simulink model "firefighting_drone_2"  (R2022b)
settings: Solver=FixedStepAuto  StartTime=0.0  StopTime=80  FixedStep=0.1  RelTol=1e-3
(part 1 of 4)
settings Model: Creator=User  LastModifiedBy=hugoaraujo
settings SolverCC: AlgebraicLoopSolver=TrustRegion
settings DataIOCC: ReturnWorkspaceOutputs=off
settings DebuggingCC: UnconnectedInputMsg=warning  UnconnectedOutputMsg=warning  UnconnectedLineMsg=warning  SFMachineParentedDataDiag=warning  ArithmeticOperatorsInVariantConditions=warning
settings ModelReferenceCC: EnableRefExpFcnMdlSchedulingChecks=on
settings SFSimCC: SimUseLocalCustomCode=off  CustomCodeUndefinedFunction=UseInterfaceOnly
settings RTWCC: RTWUseLocalCustomCode=off  DLArmComputeVersion=19.05
settings CodeAppCC: StateflowObjectComments=on

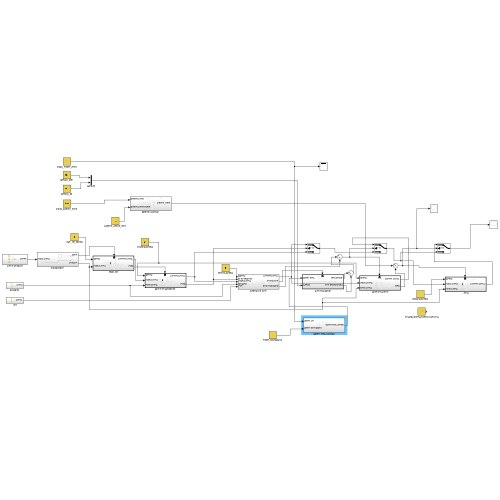
[thumbnail: Simulink's stored preview of the top-level diagram]
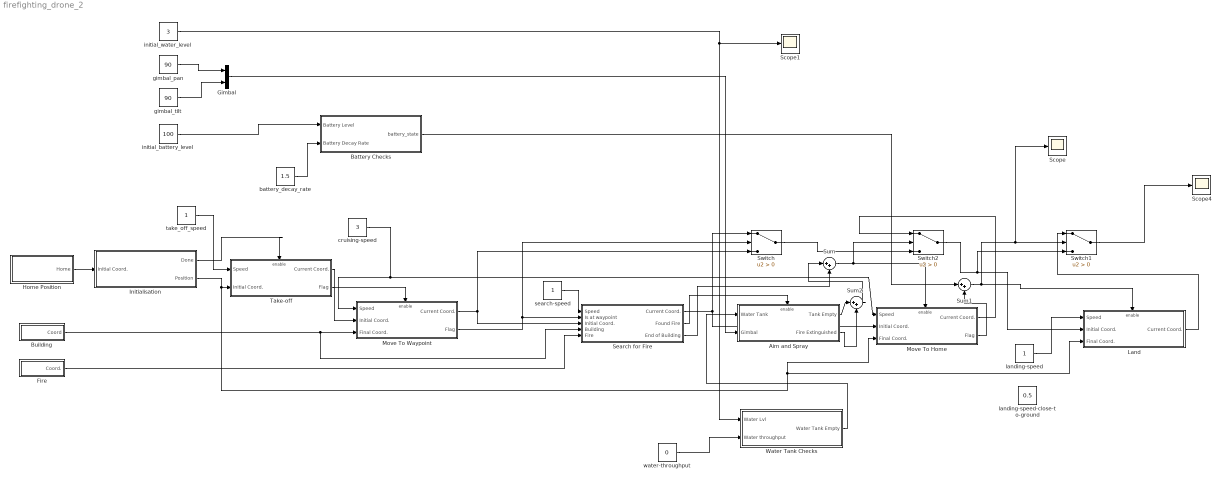
== system firefighting_drone_2 ==
  Aim and Spray : Subsystem
  Battery Checks : Subsystem
  Building : Subsystem
  Fire : Subsystem
  Gimbal : Mux  Inputs=2
  Home Position : Subsystem
  Initialisation : Subsystem
  Land : Subsystem
  Move To Home : Subsystem
  Move To Waypoint : Subsystem
  Scope : Scope
  Scope1 : Scope
  Scope4 : Scope
  Search for Fire : Subsystem
  Sum : Sum  Inputs=|++
  Sum1 : Sum  Inputs=|++
  Sum2 : Sum  Inputs=|++
  Switch : Switch  Criteria=u2 > Threshold  SaturateOnIntegerOverflow=off  InputSameDT=off
  Switch1 : Switch  Criteria=u2 > Threshold  SaturateOnIntegerOverflow=off  InputSameDT=off
  Switch2 : Switch  Criteria=u2 > Threshold  SaturateOnIntegerOverflow=off  InputSameDT=off
  Take-off : Subsystem
  Water Tank Checks : Subsystem
  battery_decay_rate : Constant  Value=1.5
  cruising-speed : Constant  Value=3
  gimbal_pan : Constant  Value=90
  gimbal_tilt : Constant  Value=90
  initial_battery_level : Constant  Value=100
  initial_water_level : Constant  Value=3
  landing-speed : Constant
  landing-speed-close-to-ground : Constant  Value=0.5
  search-speed : Constant
  take_off_speed : Constant
  water-throughput : Constant  Value=0
  wires:
  Building/1(Coord) -> Search for Fire/4(Building), Move To Waypoint/3(Final Coord.)
  cruising-speed/1 -> Move To Waypoint/1(Speed), Move To Home/1(Speed)
  Move To Waypoint/2(Flag) -> Switch/2, Search for Fire/2(Is at waypoint)
  Move To Waypoint/1(Current Coord.) -> Search for Fire/3(Initial Coord.), Switch/3
  Sum/1 -> Move To Home/Enable, Switch2/2
  Switch/1 -> Switch2/3
  Move To Home/1(Current Coord.) -> Switch2/1
  Take-off/2(Flag) -> Move To Waypoint/Enable
  Take-off/1(Current Coord.) -> Move To Waypoint/2(Initial Coord.)
  battery_decay_rate/1 -> Battery Checks/2(Battery Decay Rate)
  initial_battery_level/1 -> Battery Checks/1(Battery Level)
  gimbal_pan/1 -> Gimbal/1
  gimbal_tilt/1 -> Gimbal/2
  Battery Checks/1(battery_state) -> Sum1/1
  Move To Home/2(Flag) -> Sum1/2
  Sum1/1 -> Land/Enable, Scope/1, Switch1/2
  Initialisation/2(Position) -> Move To Home/3(Final Coord.), Land/3(Final Coord.), Take-off/2(Initial Coord.)
  Search for Fire/1(Current Coord.) -> Move To Home/2(Initial Coord.), Switch/1
  Fire/1(Coord.) -> Search for Fire/5(Fire)
  Search for Fire/2(Found Fire) -> Aim and Spray/Enable
  Search for Fire/3(End of Building) -> Sum/2
  Initialisation/1(Done) -> Take-off/Enable
  Home Position/1(Home) -> Initialisation/1(Initial Coord.)
  search-speed/1 -> Search for Fire/1(Speed)
  Switch2/1 -> Land/2(Initial Coord.), Switch1/3
  landing-speed/1 -> Land/1(Speed)
  Water Tank Checks/1(Water Tank Empty) -> Aim and Spray/1(Water Tank)
  Gimbal/1 -> Aim and Spray/2(Gimbal)
  initial_water_level/1 -> Scope1/1, Water Tank Checks/1(Water Lvl)
  Land/1(Current Coord.) -> Switch1/1
  Switch1/1 -> Scope4/1
  take_off_speed/1 -> Take-off/1(Speed)
  water-throughput/1 -> Water Tank Checks/2(Water throughput)
  Aim and Spray/2(Fire Extinguished) -> Sum2/2
  Aim and Spray/1(Tank Empty) -> Sum2/1
  Sum2/1 -> Sum/1

== system firefighting_drone_2/Aim and Spray ==
  Water Tank : Inport
  Gimbal : Inport  Port=2
  Enable : EnablePort
  Tank Empty : Outport
  Fire Extinguished : Outport  Port=2
  wires:
  Water Tank/1 -> Fire Extinguished/1, Tank Empty/1

== system firefighting_drone_2/Battery Checks ==
  Battery Level : Inport
  Battery Decay Rate : Inport  Port=2
  Constant : Constant  Value=0
  Constant1 : Constant  Value=2
  Constant2 : Constant
  If : If  IfExpression=u1 > 30  ElseIfExpressions=u1 > 15
  If Action Subsystem : Subsystem  TreatAsAtomicUnit=on
  If Action Subsystem1 : Subsystem  TreatAsAtomicUnit=on
  If Action Subsystem2 : Subsystem  TreatAsAtomicUnit=on
  Integrator : Integrator
  Merge : Merge  Inputs=3
  Scope : Scope
  Scope1 : Scope
  Sum2 : Sum  Inputs=|+-
  battery_state : Outport
  wires:
  Battery Decay Rate/1 -> Integrator/1
  Integrator/1 -> Sum2/2
  Battery Level/1 -> Sum2/1
  Sum2/1 -> Scope1/1, If/1
  Constant1/1 -> If Action Subsystem1/1(In1)
  If/1 -> If Action Subsystem/Action
  Constant/1 -> If Action Subsystem/1(In1)
  If Action Subsystem/1(Out1) -> Merge/1
  If Action Subsystem1/1(Out1) -> Merge/3
  Merge/1 -> Scope/1, battery_state/1
  If/3 -> If Action Subsystem1/Action
  Constant2/1 -> If Action Subsystem2/1(In1)
  If/2 -> If Action Subsystem2/Action
  If Action Subsystem2/1(Out1) -> Merge/2

== system firefighting_drone_2/Building ==
  Building.x : Constant  Value=25
  Building.y : Constant  Value=15
  Building.z : Constant  Value=2
  Mux : Mux  Inputs=3
  Coord : Outport  VectorParamsAs1DForOutWhenUnconnected=off
  wires:
  Building.y/1 -> Mux/2
  Building.z/1 -> Mux/3
  Building.x/1 -> Mux/1
  Mux/1 -> Coord/1

== system firefighting_drone_2/Fire ==
  Fire.x : Constant  Value=25
  Fire.y : Constant  Value=20
  Fire.z : Constant  Value=12
  Mux : Mux  Inputs=3
  Coord. : Outport  VectorParamsAs1DForOutWhenUnconnected=off
  wires:
  Fire.y/1 -> Mux/2
  Fire.z/1 -> Mux/3
  Fire.x/1 -> Mux/1
  Mux/1 -> Coord./1

== system firefighting_drone_2/Home Position ==
  Home.x : Constant  Value=0
  Home.y : Constant  Value=0
  Home.z : Constant  Value=0
  Mux : Mux  Inputs=3
  Home : Outport  VectorParamsAs1DForOutWhenUnconnected=off
  wires:
  Home.x/1 -> Mux/1
  Home.y/1 -> Mux/2
  Home.z/1 -> Mux/3
  Mux/1 -> Home/1

== system firefighting_drone_2/Initialisation ==
  Initial Coord. : Inport
  Constant : Constant
  Done : Outport  VectorParamsAs1DForOutWhenUnconnected=off
  Position : Outport  Port=2  VectorParamsAs1DForOutWhenUnconnected=off
  wires:
  Initial Coord./1 -> Position/1
  Constant/1 -> Done/1

== system firefighting_drone_2/Land ==
  Speed : Inport
  Initial Coord. : Inport  Port=2
  Final Coord. : Inport  Port=3
  Enable : EnablePort
  Constant : Constant
  Constant1 : Constant  Value=0
  Demux : Demux  Outputs=3
  Demux1 : Demux  Outputs=3
  Display : Display
  Display2 : Display
  Move Arm1 : Subsystem
  Move Arm2 : Subsystem
  Move Arm3 : Subsystem
  Mux : Mux  Inputs=3
  Mux1 : Mux  Inputs=3
  Scope : Scope
  Scope1 : Scope  NumInputPorts=3
  Scope2 : Scope
  Scope3 : Scope
  Sum : Sum  Inputs=3
  Switch : Switch  Threshold=3  SaturateOnIntegerOverflow=off  InputSameDT=off
  Current Coord. : Outport  VectorParamsAs1DForOutWhenUnconnected=off
  wires:
  Demux1/1 -> Mux1/1, Scope3/1, Move Arm1/3(Desired Angle)
  Demux/1 -> Scope2/1, Move Arm1/2(Starting Angle)
  Move Arm3/1(Out1) -> Scope1/3, Mux/3  "Z"
  Demux/2 -> Move Arm2/2(Starting Angle)
  Speed/1 -> Move Arm2/1(Angular Accel), Move Arm3/1(Angular Accel), Move Arm1/1(Angular Accel)
  Move Arm2/1(Out1) -> Mux/2, Scope1/2  "Y"
  Move Arm1/1(Out1) -> Mux/1, Scope1/1  "X"
  Demux/3 -> Move Arm3/2(Starting Angle)
  Demux1/2 -> Move Arm2/3(Desired Angle), Mux1/2
  Demux1/3 -> Move Arm3/3(Desired Angle), Mux1/3
  Mux/1 -> Display2/1, Current Coord./1, Scope/1
  Mux1/1 -> Display/1
  Initial Coord./1 -> Demux/1
  Final Coord./1 -> Demux1/1
  Move Arm3/2(Done) -> Sum/3
  Move Arm1/2(Done) -> Sum/1
  Move Arm2/2(Done) -> Sum/2
  Constant1/1 -> Switch/3
  Constant/1 -> Switch/1
  Sum/1 -> Switch/2
  Switch/1 -> ?

== system firefighting_drone_2/Move To Home ==
  Speed : Inport
  Initial Coord. : Inport  Port=2
  Final Coord. : Inport  Port=3
  Enable : EnablePort
  Constant : Constant
  Constant1 : Constant  Value=0
  Demux : Demux  Outputs=3
  Demux1 : Demux  Outputs=3
  Display : Display
  Display2 : Display
  Move Arm1 : Subsystem
  Move Arm2 : Subsystem
  Move Arm3 : Subsystem
  Mux : Mux  Inputs=3
  Mux1 : Mux  Inputs=3
  Scope : Scope
  Scope1 : Scope  NumInputPorts=3
  Scope2 : Scope
  Scope3 : Scope
  Sum : Sum  Inputs=3
  Switch : Switch  Threshold=3  SaturateOnIntegerOverflow=off  InputSameDT=off
  Current Coord. : Outport  VectorParamsAs1DForOutWhenUnconnected=off
  Flag : Outport  Port=2  VectorParamsAs1DForOutWhenUnconnected=off
  wires:
  Demux1/1 -> Mux1/1, Scope3/1, Move Arm1/3(Desired Angle)
  Demux/1 -> Scope2/1, Move Arm1/2(Starting Angle)
  Move Arm3/1(Out1) -> Scope1/3, Mux/3  "Z"
  Demux/2 -> Move Arm2/2(Starting Angle)
  Speed/1 -> Move Arm2/1(Angular Accel), Move Arm3/1(Angular Accel), Move Arm1/1(Angular Accel)
  Move Arm2/1(Out1) -> Mux/2, Scope1/2  "Y"
  Move Arm1/1(Out1) -> Mux/1, Scope1/1  "X"
  Demux/3 -> Move Arm3/2(Starting Angle)
  Demux1/2 -> Move Arm2/3(Desired Angle), Mux1/2
  Demux1/3 -> Move Arm3/3(Desired Angle), Mux1/3
  Mux/1 -> Display2/1, Current Coord./1, Scope/1
  Mux1/1 -> Display/1
  Initial Coord./1 -> Demux/1
  Final Coord./1 -> Demux1/1
  Move Arm3/2(Done) -> Sum/3
  Move Arm1/2(Done) -> Sum/1
  Move Arm2/2(Done) -> Sum/2
  Constant1/1 -> Switch/3
  Constant/1 -> Switch/1
  Sum/1 -> Switch/2
  Switch/1 -> Flag/1

== system firefighting_drone_2/Move To Waypoint ==
  Speed : Inport
  Initial Coord. : Inport  Port=2
  Final Coord. : Inport  Port=3
  Enable : EnablePort
  Constant : Constant
  Constant1 : Constant  Value=0
  Demux : Demux  Outputs=3
  Demux1 : Demux  Outputs=3
  Display : Display
  Display2 : Display
  Move X : Subsystem
  Move Y : Subsystem
  Move Z : Subsystem
  Mux : Mux  Inputs=3
  Mux1 : Mux  Inputs=3
  Scope : Scope
  Scope1 : Scope  NumInputPorts=3
  Scope2 : Scope
  Scope3 : Scope
  Sum : Sum  Inputs=3
  Switch : Switch  Threshold=3  SaturateOnIntegerOverflow=off  InputSameDT=off
  Current Coord. : Outport  VectorParamsAs1DForOutWhenUnconnected=off
  Flag : Outport  Port=2  VectorParamsAs1DForOutWhenUnconnected=off
  wires:
  Demux1/1 -> Mux1/1, Scope3/1, Move X/3(Desired Angle)
  Demux/1 -> Scope2/1, Move X/2(Starting Angle)
  Move Z/1(Out1) -> Scope1/3, Mux/3
  Demux/2 -> Move Y/2(Starting Angle)
  Speed/1 -> Move Y/1(Angular Accel), Move Z/1(Angular Accel), Move X/1(Angular Accel)
  Move Y/1(Out1) -> Mux/2, Scope1/2
  Move X/1(Out1) -> Mux/1, Scope1/1
  Demux/3 -> Move Z/2(Starting Angle)
  Demux1/2 -> Move Y/3(Desired Angle), Mux1/2
  Demux1/3 -> Move Z/3(Desired Angle), Mux1/3
  Mux/1 -> Display2/1, Current Coord./1, Scope/1
  Mux1/1 -> Display/1
  Initial Coord./1 -> Demux/1
  Final Coord./1 -> Demux1/1
  Move Z/2(Done) -> Sum/3
  Move X/2(Done) -> Sum/1
  Move Y/2(Done) -> Sum/2
  Constant1/1 -> Switch/3
  Constant/1 -> Switch/1
  Sum/1 -> Switch/2
  Switch/1 -> Flag/1

== system firefighting_drone_2/Search for Fire ==
  Speed : Inport
  Is at waypoint : Inport  Port=2
  Initial Coord. : Inport  Port=3
  Building : Inport  Port=4
  Fire : Inport  Port=5
  Scope : Scope
  Seaerch-fire : Subsystem
  Current Coord. : Outport
  Found Fire : Outport  Port=2
  End of Building : Outport  Port=3
  wires:
  Seaerch-fire/3(Flag1) -> End of Building/1
  Seaerch-fire/2(Flag) -> Scope/1, Found Fire/1
  Seaerch-fire/1(Current Coord.) -> Current Coord./1
  Building/1 -> Seaerch-fire/4(Building)
  Is at waypoint/1 -> Seaerch-fire/Enable
  Fire/1 -> Seaerch-fire/3(Fire)
  Speed/1 -> Seaerch-fire/1(Speed)
  Initial Coord./1 -> Seaerch-fire/2(Initial Coord.)

== system firefighting_drone_2/Take-off ==
  Speed : Inport
  Initial Coord. : Inport  Port=2
  Enable : EnablePort
  Constant : Constant
  Constant1 : Constant  Value=0
  CoordX : Subsystem
  CoordY : Subsystem
  CoordZ : Subsystem
  Demux : Demux  Outputs=3
  Demux1 : Demux  Outputs=3
  Display : Display
  Display2 : Display
  Mux : Mux  Inputs=3
  Mux1 : Mux  Inputs=3
  Scope : Scope
  Scope1 : Scope  NumInputPorts=3
  Scope2 : Scope
  Scope3 : Scope
  Sum : Sum  Inputs=3
  Switch : Switch  Threshold=3  SaturateOnIntegerOverflow=off  InputSameDT=off
  Take-off Height : Subsystem
  Current Coord. : Outport  VectorParamsAs1DForOutWhenUnconnected=off
  Flag : Outport  Port=2  VectorParamsAs1DForOutWhenUnconnected=off
  wires:
  Demux1/1 -> Mux1/1, Scope3/1, CoordX/3(Desired Angle)
  Demux/1 -> Scope2/1, CoordX/2(Starting Angle)
  CoordZ/1(Out1) -> Scope1/3, Mux/3
  Demux/2 -> CoordY/2(Starting Angle)
  Speed/1 -> CoordY/1(Angular Accel), CoordZ/1(Angular Accel), CoordX/1(Angular Accel)
  CoordY/1(Out1) -> Mux/2, Scope1/2
  CoordX/1(Out1) -> Mux/1, Scope1/1
  Demux/3 -> CoordZ/2(Starting Angle)
  Demux1/2 -> CoordY/3(Desired Angle), Mux1/2
  Demux1/3 -> CoordZ/3(Desired Angle), Mux1/3
  Mux/1 -> Display2/1, Current Coord./1, Scope/1
  Mux1/1 -> Display/1
  Initial Coord./1 -> Demux/1
  Take-off Height/1(Coord) -> Demux1/1
  CoordZ/2(Done) -> Sum/3
  CoordX/2(Done) -> Sum/1
  CoordY/2(Done) -> Sum/2
  Constant1/1 -> Switch/3
  Constant/1 -> Switch/1
  Sum/1 -> Switch/2
  Switch/1 -> Flag/1

== system firefighting_drone_2/Water Tank Checks ==
  Water Lvl : Inport
  Water throughput : Inport  Port=2
  Constant2 : Constant  Value=0
  Constant3 : Constant
  If Action Subsystem : Subsystem  TreatAsAtomicUnit=on
  If Action Subsystem1 : Subsystem  TreatAsAtomicUnit=on
  If1 : If  IfExpression=u1 > 15
  Integrator : Integrator
  Merge : Merge
  Scope : Scope
  Sum2 : Sum  Inputs=|+-
  Water Tank Empty : Outport
  wires:
  Water throughput/1 -> Integrator/1
  Integrator/1 -> Sum2/2
  Water Lvl/1 -> Sum2/1
  Sum2/1 -> Scope/1, If1/1
  If Action Subsystem1/1(Out1) -> Merge/2
  Constant3/1 -> If Action Subsystem1/1(In1)
  Constant2/1 -> If Action Subsystem/1(In1)
  If1/1 -> If Action Subsystem/Action
  If Action Subsystem/1(Out1) -> Merge/1
  Merge/1 -> Water Tank Empty/1
  If1/2 -> If Action Subsystem1/Action

== system firefighting_drone_2/Battery Checks/If Action Subsystem ==
  In1 : Inport
  Action Port : ActionPort  ActionPortLabel=if(u1 > 30)
  Out1 : Outport
  wires:
  In1/1 -> Out1/1

== system firefighting_drone_2/Battery Checks/If Action Subsystem1 ==
  In1 : Inport
  Action Port : ActionPort  ActionPortLabel=else
  Out1 : Outport
  wires:
  In1/1 -> Out1/1

== system firefighting_drone_2/Battery Checks/If Action Subsystem2 ==
  In1 : Inport
  Action Port : ActionPort  ActionPortLabel=elseif(u1 > 15)
  Out1 : Outport
  wires:
  In1/1 -> Out1/1

== system firefighting_drone_2/Land/Move Arm1 ==
  Angular Accel : Inport
  Starting Angle : Inport  Port=2
  Desired Angle : Inport  Port=3
  If : If
  If Action Subsystem : Subsystem  TreatAsAtomicUnit=on
  If Action Subsystem1 : Subsystem  TreatAsAtomicUnit=on
  Integrator1 : Integrator
  Scope : Scope
  Scope1 : Scope
  Subsystem : Subsystem
  Sum1 : Sum  Inputs=|++
  Sum2 : Sum  Inputs=|+-
  Sum3 : Sum  Inputs=|-+
  Switch : Switch  Criteria=u2 ~= 0  SaturateOnIntegerOverflow=off  InputSameDT=off
  Out1 : Outport  VectorParamsAs1DForOutWhenUnconnected=off
  Done : Outport  Port=2  VectorParamsAs1DForOutWhenUnconnected=off
  wires:
  Angular Accel/1 -> Integrator1/1
  If Action Subsystem/1(Out1) -> Switch/3
  Sum2/1 -> If/1
  If/2 -> If Action Subsystem1/Action
  Starting Angle/1 -> Sum2/2, Sum3/2, Sum1/2
  Desired Angle/1 -> Scope1/1, Subsystem/1(Desired Angle), Sum2/1
  If Action Subsystem1/1(Out1) -> Switch/1, Switch/2
  If/1 -> If Action Subsystem/Action
  Integrator1/1 -> Sum1/1, Sum3/1
  Sum3/1 -> If Action Subsystem1/1(In1)
  Sum1/1 -> If Action Subsystem/1(In1)
  Switch/1 -> Subsystem/2(Current Angle)
  Subsystem/1(Out1) -> Scope/1, Out1/1
  Subsystem/2(Done) -> Done/1

== system firefighting_drone_2/Land/Move Arm2 ==
  Angular Accel : Inport
  Starting Angle : Inport  Port=2
  Desired Angle : Inport  Port=3
  If : If
  If Action Subsystem : Subsystem  TreatAsAtomicUnit=on
  If Action Subsystem1 : Subsystem  TreatAsAtomicUnit=on
  Integrator1 : Integrator
  Scope : Scope
  Subsystem : Subsystem
  Sum1 : Sum  Inputs=|++
  Sum2 : Sum  Inputs=|+-
  Sum3 : Sum  Inputs=|-+
  Switch : Switch  Criteria=u2 ~= 0  SaturateOnIntegerOverflow=off  InputSameDT=off
  Out1 : Outport  VectorParamsAs1DForOutWhenUnconnected=off
  Done : Outport  Port=2  VectorParamsAs1DForOutWhenUnconnected=off
  wires:
  Angular Accel/1 -> Integrator1/1
  If Action Subsystem/1(Out1) -> Switch/3
  Sum2/1 -> If/1
  If/2 -> If Action Subsystem1/Action
  Starting Angle/1 -> Sum2/2, Sum3/2, Sum1/2
  Desired Angle/1 -> Subsystem/1(Desired Angle), Sum2/1
  If Action Subsystem1/1(Out1) -> Switch/1, Switch/2
  If/1 -> If Action Subsystem/Action
  Integrator1/1 -> Sum1/1, Sum3/1
  Sum3/1 -> If Action Subsystem1/1(In1)
  Sum1/1 -> If Action Subsystem/1(In1)
  Switch/1 -> Subsystem/2(Current Angle)
  Subsystem/1(Out1) -> Scope/1, Out1/1
  Subsystem/2(Done) -> Done/1

== system firefighting_drone_2/Land/Move Arm3 ==
  Angular Accel : Inport
  Starting Angle : Inport  Port=2
  Desired Angle : Inport  Port=3
  If : If
  If Action Subsystem : Subsystem  TreatAsAtomicUnit=on
  If Action Subsystem1 : Subsystem  TreatAsAtomicUnit=on
  Integrator1 : Integrator
  Scope : Scope
  Subsystem : Subsystem
  Sum1 : Sum  Inputs=|++
  Sum2 : Sum  Inputs=|+-
  Sum3 : Sum  Inputs=|-+
  Switch : Switch  Criteria=u2 ~= 0  SaturateOnIntegerOverflow=off  InputSameDT=off
  Out1 : Outport  VectorParamsAs1DForOutWhenUnconnected=off
  Done : Outport  Port=2  VectorParamsAs1DForOutWhenUnconnected=off
  wires:
  Angular Accel/1 -> Integrator1/1
  If Action Subsystem/1(Out1) -> Switch/3
  Sum2/1 -> If/1
  If/2 -> If Action Subsystem1/Action
  Starting Angle/1 -> Sum2/2, Sum3/2, Sum1/2
  Desired Angle/1 -> Subsystem/1(Desired Angle), Sum2/1
  If Action Subsystem1/1(Out1) -> Switch/1, Switch/2
  If/1 -> If Action Subsystem/Action
  Integrator1/1 -> Sum1/1, Sum3/1
  Sum3/1 -> If Action Subsystem1/1(In1)
  Sum1/1 -> If Action Subsystem/1(In1)
  Switch/1 -> Subsystem/2(Current Angle)
  Subsystem/1(Out1) -> Scope/1, Out1/1
  Subsystem/2(Done) -> Done/1

== system firefighting_drone_2/Move To Home/Move Arm1 ==
  Angular Accel : Inport
  Starting Angle : Inport  Port=2
  Desired Angle : Inport  Port=3
  If : If
  If Action Subsystem : Subsystem  TreatAsAtomicUnit=on
  If Action Subsystem1 : Subsystem  TreatAsAtomicUnit=on
  Integrator1 : Integrator
  Scope : Scope
  Scope1 : Scope
  Subsystem : Subsystem
  Sum1 : Sum  Inputs=|++
  Sum2 : Sum  Inputs=|+-
  Sum3 : Sum  Inputs=|-+
  Switch : Switch  Criteria=u2 ~= 0  SaturateOnIntegerOverflow=off  InputSameDT=off
  Out1 : Outport  VectorParamsAs1DForOutWhenUnconnected=off
  Done : Outport  Port=2  VectorParamsAs1DForOutWhenUnconnected=off
  wires:
  Angular Accel/1 -> Integrator1/1
  If Action Subsystem/1(Out1) -> Switch/3
  Sum2/1 -> If/1
  If/2 -> If Action Subsystem1/Action
  Starting Angle/1 -> Sum2/2, Sum3/2, Sum1/2
  Desired Angle/1 -> Scope1/1, Subsystem/1(Desired Angle), Sum2/1
  If Action Subsystem1/1(Out1) -> Switch/1, Switch/2
  If/1 -> If Action Subsystem/Action
  Integrator1/1 -> Sum1/1, Sum3/1
  Sum3/1 -> If Action Subsystem1/1(In1)
  Sum1/1 -> If Action Subsystem/1(In1)
  Switch/1 -> Subsystem/2(Current Angle)
  Subsystem/1(Out1) -> Scope/1, Out1/1
  Subsystem/2(Done) -> Done/1

== system firefighting_drone_2/Move To Home/Move Arm2 ==
  Angular Accel : Inport
  Starting Angle : Inport  Port=2
  Desired Angle : Inport  Port=3
  If : If
  If Action Subsystem : Subsystem  TreatAsAtomicUnit=on
  If Action Subsystem1 : Subsystem  TreatAsAtomicUnit=on
  Integrator1 : Integrator
  Scope : Scope
  Subsystem : Subsystem
  Sum1 : Sum  Inputs=|++
  Sum2 : Sum  Inputs=|+-
  Sum3 : Sum  Inputs=|-+
  Switch : Switch  Criteria=u2 ~= 0  SaturateOnIntegerOverflow=off  InputSameDT=off
  Out1 : Outport  VectorParamsAs1DForOutWhenUnconnected=off
  Done : Outport  Port=2  VectorParamsAs1DForOutWhenUnconnected=off
  wires:
  Angular Accel/1 -> Integrator1/1
  If Action Subsystem/1(Out1) -> Switch/3
  Sum2/1 -> If/1
  If/2 -> If Action Subsystem1/Action
  Starting Angle/1 -> Sum2/2, Sum3/2, Sum1/2
  Desired Angle/1 -> Subsystem/1(Desired Angle), Sum2/1
  If Action Subsystem1/1(Out1) -> Switch/1, Switch/2
  If/1 -> If Action Subsystem/Action
  Integrator1/1 -> Sum1/1, Sum3/1
  Sum3/1 -> If Action Subsystem1/1(In1)
  Sum1/1 -> If Action Subsystem/1(In1)
  Switch/1 -> Subsystem/2(Current Angle)
  Subsystem/1(Out1) -> Scope/1, Out1/1
  Subsystem/2(Done) -> Done/1

== system firefighting_drone_2/Move To Home/Move Arm3 ==
  Angular Accel : Inport
  Starting Angle : Inport  Port=2
  Desired Angle : Inport  Port=3
  If : If
  If Action Subsystem : Subsystem  TreatAsAtomicUnit=on
  If Action Subsystem1 : Subsystem  TreatAsAtomicUnit=on
  Integrator1 : Integrator
  Scope : Scope
  Subsystem : Subsystem
  Sum1 : Sum  Inputs=|++
  Sum2 : Sum  Inputs=|+-
  Sum3 : Sum  Inputs=|-+
  Switch : Switch  Criteria=u2 ~= 0  SaturateOnIntegerOverflow=off  InputSameDT=off
  Out1 : Outport  VectorParamsAs1DForOutWhenUnconnected=off
  Done : Outport  Port=2  VectorParamsAs1DForOutWhenUnconnected=off
  wires:
  Angular Accel/1 -> Integrator1/1
  If Action Subsystem/1(Out1) -> Switch/3
  Sum2/1 -> If/1
  If/2 -> If Action Subsystem1/Action
  Starting Angle/1 -> Sum2/2, Sum3/2, Sum1/2
  Desired Angle/1 -> Subsystem/1(Desired Angle), Sum2/1
  If Action Subsystem1/1(Out1) -> Switch/1, Switch/2
  If/1 -> If Action Subsystem/Action
  Integrator1/1 -> Sum1/1, Sum3/1
  Sum3/1 -> If Action Subsystem1/1(In1)
  Sum1/1 -> If Action Subsystem/1(In1)
  Switch/1 -> Subsystem/2(Current Angle)
  Subsystem/1(Out1) -> Scope/1, Out1/1
  Subsystem/2(Done) -> Done/1

== system firefighting_drone_2/Move To Waypoint/Move X ==
  Angular Accel : Inport
  Starting Angle : Inport  Port=2
  Desired Angle : Inport  Port=3
  If : If
  If Action Subsystem : Subsystem  TreatAsAtomicUnit=on
  If Action Subsystem1 : Subsystem  TreatAsAtomicUnit=on
  Integrator1 : Integrator
  Scope : Scope
  Scope1 : Scope
  Subsystem : Subsystem
  Sum1 : Sum  Inputs=|++
  Sum2 : Sum  Inputs=|+-
  Sum3 : Sum  Inputs=|-+
  Switch : Switch  Criteria=u2 ~= 0  SaturateOnIntegerOverflow=off  InputSameDT=off
  Out1 : Outport  VectorParamsAs1DForOutWhenUnconnected=off
  Done : Outport  Port=2  VectorParamsAs1DForOutWhenUnconnected=off
  wires:
  Angular Accel/1 -> Integrator1/1
  If Action Subsystem/1(Out1) -> Switch/3
  Sum2/1 -> If/1
  If/2 -> If Action Subsystem1/Action
  Starting Angle/1 -> Sum2/2, Sum3/2, Sum1/2
  Desired Angle/1 -> Scope1/1, Subsystem/1(Desired Angle), Sum2/1
  If Action Subsystem1/1(Out1) -> Switch/1, Switch/2
  If/1 -> If Action Subsystem/Action
  Integrator1/1 -> Sum1/1, Sum3/1
  Sum3/1 -> If Action Subsystem1/1(In1)
  Sum1/1 -> If Action Subsystem/1(In1)
  Switch/1 -> Subsystem/2(Current Angle)
  Subsystem/1(Out1) -> Scope/1, Out1/1
  Subsystem/2(Done) -> Done/1

== system firefighting_drone_2/Move To Waypoint/Move Y ==
  Angular Accel : Inport
  Starting Angle : Inport  Port=2
  Desired Angle : Inport  Port=3
  If : If
  If Action Subsystem : Subsystem  TreatAsAtomicUnit=on
  If Action Subsystem1 : Subsystem  TreatAsAtomicUnit=on
  Integrator1 : Integrator
  Scope : Scope
  Subsystem : Subsystem
  Sum1 : Sum  Inputs=|++
  Sum2 : Sum  Inputs=|+-
  Sum3 : Sum  Inputs=|-+
  Switch : Switch  Criteria=u2 ~= 0  SaturateOnIntegerOverflow=off  InputSameDT=off
  Out1 : Outport  VectorParamsAs1DForOutWhenUnconnected=off
  Done : Outport  Port=2  VectorParamsAs1DForOutWhenUnconnected=off
  wires:
  Angular Accel/1 -> Integrator1/1
  If Action Subsystem/1(Out1) -> Switch/3
  Sum2/1 -> If/1
  If/2 -> If Action Subsystem1/Action
  Starting Angle/1 -> Sum2/2, Sum3/2, Sum1/2
  Desired Angle/1 -> Subsystem/1(Desired Angle), Sum2/1
  If Action Subsystem1/1(Out1) -> Switch/1, Switch/2
  If/1 -> If Action Subsystem/Action
  Integrator1/1 -> Sum1/1, Sum3/1
  Sum3/1 -> If Action Subsystem1/1(In1)
  Sum1/1 -> If Action Subsystem/1(In1)
  Switch/1 -> Subsystem/2(Current Angle)
  Subsystem/1(Out1) -> Scope/1, Out1/1
  Subsystem/2(Done) -> Done/1

== system firefighting_drone_2/Move To Waypoint/Move Z ==
  Angular Accel : Inport
  Starting Angle : Inport  Port=2
  Desired Angle : Inport  Port=3
  If : If
  If Action Subsystem : Subsystem  TreatAsAtomicUnit=on
  If Action Subsystem1 : Subsystem  TreatAsAtomicUnit=on
  Integrator1 : Integrator
  Scope : Scope
  Subsystem : Subsystem
  Sum1 : Sum  Inputs=|++
  Sum2 : Sum  Inputs=|+-
  Sum3 : Sum  Inputs=|-+
  Switch : Switch  Criteria=u2 ~= 0  SaturateOnIntegerOverflow=off  InputSameDT=off
  Out1 : Outport  VectorParamsAs1DForOutWhenUnconnected=off
  Done : Outport  Port=2  VectorParamsAs1DForOutWhenUnconnected=off
  wires:
  Angular Accel/1 -> Integrator1/1
  If Action Subsystem/1(Out1) -> Switch/3
  Sum2/1 -> If/1
  If/2 -> If Action Subsystem1/Action
  Starting Angle/1 -> Sum2/2, Sum3/2, Sum1/2
  Desired Angle/1 -> Subsystem/1(Desired Angle), Sum2/1
  If Action Subsystem1/1(Out1) -> Switch/1, Switch/2
  If/1 -> If Action Subsystem/Action
  Integrator1/1 -> Sum1/1, Sum3/1
  Sum3/1 -> If Action Subsystem1/1(In1)
  Sum1/1 -> If Action Subsystem/1(In1)
  Switch/1 -> Subsystem/2(Current Angle)
  Subsystem/1(Out1) -> Scope/1, Out1/1
  Subsystem/2(Done) -> Done/1

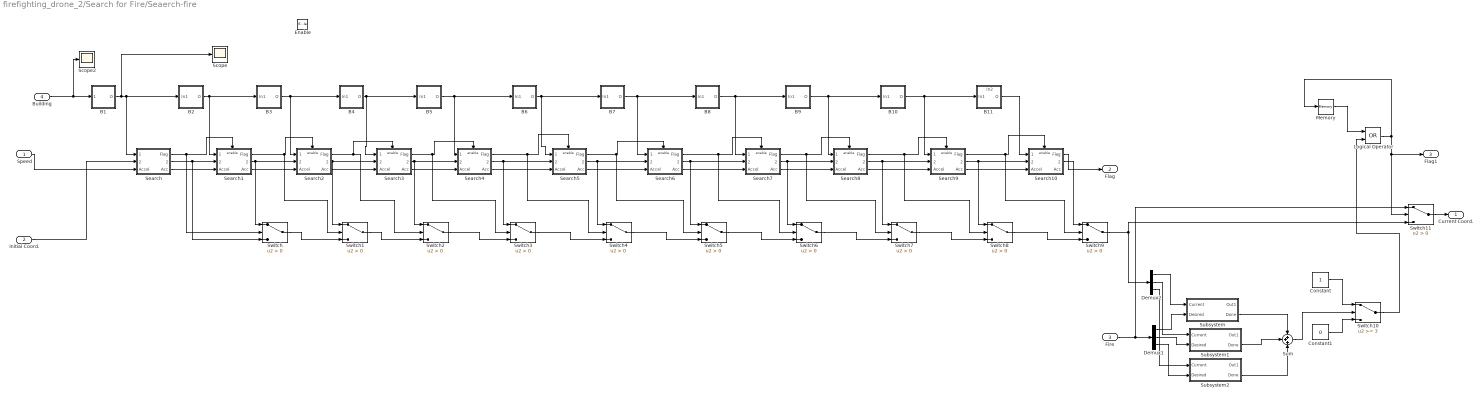
== system firefighting_drone_2/Search for Fire/Seaerch-fire ==
  Speed : Inport
  Initial Coord. : Inport  Port=2
  Fire : Inport  Port=3
  Building : Inport  Port=4
  Enable : EnablePort
  B1 : Subsystem
  B10 : Subsystem
  B11 : Subsystem
      settings: PortSchema="{\"entries\":[{\"content\":{\"sides\":[{\"content\":{\"connectorIds\":[\"In1\"]},\"type\":\"ConnectorPlacement.EquallySpacedRectSide\",\"uuid\":\"e2f7b148-e440-4145-b7d1-8438cbf5f998\"},{\"content\":{\"connectorIds\":[\"Out1\"],\"side\":\"RIGHT\"},\"type\":\"ConnectorPlacement.EquallySpacedRectSide\",\"uuid\":\"cb40fe30-092c-4751-a9fe-c202a7344311\"},{\"content\":{\"connectorIds\":[\"In2\"],\"side\":\"TOP\"},\"type\":\"ConnectorPlacement.EquallySpacedRectSide\",\"uuid\":\"468bd48b-21e5-4b86-968a-118d18909670\"}]},\"type\":\"ConnectorPlacement.EquallySpacedConnector\",\"uuid\":\"093b63ec-163d-49d6-85c2-7237e7cb80b7\"}],\"packageUris\":[\"http://schema.mathworks.com/mf0/Connector/R2020b\"],\"version\":\"1.0\"}"
  B2 : Subsystem
  B3 : Subsystem
  B4 : Subsystem
  B5 : Subsystem
  B6 : Subsystem
  B7 : Subsystem
  B8 : Subsystem
  B9 : Subsystem
  Constant : Constant
  Constant1 : Constant  Value=0
  Demux1 : Demux  Outputs=3
  Demux2 : Demux  Outputs=3
  Logical Operator : Logic  Operator=OR  AllPortsSameDT=off  OutDataTypeStr=boolean
  Memory : Memory
  Scope : Scope
  Scope2 : Scope
  Search : Subsystem
  Search1 : Subsystem
  Search10 : Subsystem
  Search2 : Subsystem
  Search3 : Subsystem
  Search4 : Subsystem
  Search5 : Subsystem
  Search6 : Subsystem
  Search7 : Subsystem
  Search8 : Subsystem
  Search9 : Subsystem
  Subsystem : Subsystem
  Subsystem1 : Subsystem
  Subsystem2 : Subsystem
  Sum : Sum  Inputs=3
  Switch{,1..9,11} (11 alike) : Switch  Criteria=u2 > Threshold  SaturateOnIntegerOverflow=off  InputSameDT=off
  Switch10 : Switch  Threshold=3  SaturateOnIntegerOverflow=off  InputSameDT=off
  Current Coord. : Outport  VectorParamsAs1DForOutWhenUnconnected=off
  Flag : Outport  Port=2  VectorParamsAs1DForOutWhenUnconnected=off
  Flag1 : Outport  Port=3  VectorParamsAs1DForOutWhenUnconnected=off
  wires:
  Building/1 -> Scope2/1, B1/1(Building)
  B1/1(O) -> Scope/1, B2/1(In1), Search/1(Final Coord.)
  B2/1(O) -> Search1/1(Final Coord.), B3/1(In1)
  B4/1(O) -> Search3/1(Final Coord.), B5/1(In1)
  B3/1(O) -> Search2/1(Final Coord.), B4/1(In1)
  B6/1(O) -> Search5/1(Final Coord.), B7/1(In1)
  B8/1(O) -> Search7/1(Final Coord.), B9/1(In1)
  B5/1(O) -> Search4/1(Final Coord.), B6/1(In1)
  B7/1(O) -> Search6/1(Final Coord.), B8/1(In1)
  B10/1(O) -> Search9/1(Final Coord.), B11/1(In1)
  B9/1(O) -> Search8/1(Final Coord.), B10/1(In1)
  Speed/1 -> Search/3(Accel)
  Search/2(Current Coord.) -> Switch/3, Search1/2(Initial Coord.)
  Search/3(Acc) -> Search1/3(Accel)
  Search/1(Flag) -> Switch/2, Search1/Enable
  Search1/2(Current Coord.) -> Search2/2(Initial Coord.), Switch/1
  Search1/3(Acc) -> Search2/3(Accel)
  Search1/1(Flag) -> Search2/Enable, Switch1/2
  Search2/1(Flag) -> Switch2/2, Search3/Enable
  Search2/2(Current Coord.) -> Search3/2(Initial Coord.), Switch1/1
  Search2/3(Acc) -> Search3/3(Accel)
  Search3/2(Current Coord.) -> Switch2/1, Search4/2(Initial Coord.)
  Search3/3(Acc) -> Search4/3(Accel)
  Search3/1(Flag) -> Search4/Enable, Switch3/2
  Search4/3(Acc) -> Search5/3(Accel)
  Search4/1(Flag) -> Search5/Enable, Switch4/2
  Search5/2(Current Coord.) -> Search6/2(Initial Coord.), Switch4/1
  Search5/3(Acc) -> Search6/3(Accel)
  Search5/1(Flag) -> Search6/Enable, Switch5/2
  Search6/1(Flag) -> Search7/Enable, Switch6/2
  Search6/2(Current Coord.) -> Search7/2(Initial Coord.), Switch5/1
  Search6/3(Acc) -> Search7/3(Accel)
  Search7/1(Flag) -> Search8/Enable, Switch7/2
  Search7/2(Current Coord.) -> Search8/2(Initial Coord.), Switch6/1
  Search7/3(Acc) -> Search8/3(Accel)
  Search8/2(Current Coord.) -> Search9/2(Initial Coord.), Switch7/1
  Search8/3(Acc) -> Search9/3(Accel)
  Search8/1(Flag) -> Search9/Enable, Switch8/2
  Search9/1(Flag) -> Search10/Enable, Switch9/2
  B11/1(O) -> Search10/1(Final Coord.)
  Search9/2(Current Coord.) -> Search10/2(Initial Coord.), Switch8/1
  Search9/3(Acc) -> Search10/3(Accel)
  Switch/1 -> Switch1/3
  Switch1/1 -> Switch2/3
  Switch2/1 -> Switch3/3
  Search4/2(Current Coord.) -> Search5/2(Initial Coord.), Switch3/1
  Switch3/1 -> Switch4/3
  Switch4/1 -> Switch5/3
  Switch5/1 -> Switch6/3
  Switch6/1 -> Switch7/3
  Switch7/1 -> Switch8/3
  Switch8/1 -> Switch9/3
  Search10/2(Current Coord.) -> Switch9/1
  Search10/1(Flag) -> Flag/1
  Initial Coord./1 -> Search/2(Initial Coord.)
  Switch9/1 -> Demux2/1, Switch11/3
  Demux1/1 -> Subsystem/2("Desired ")
  Demux2/1 -> Subsystem/1("Current ")
  Demux2/2 -> Subsystem1/1("Current ")
  Demux2/3 -> Subsystem2/1("Current ")
  Demux1/2 -> Subsystem1/2("Desired ")
  Demux1/3 -> Subsystem2/2("Desired ")
  Constant1/1 -> Switch10/3
  Sum/1 -> Switch10/2
  Switch10/1 -> Logical Operator/2
  Constant/1 -> Switch10/1
  Subsystem/2(Done) -> Sum/1
  Subsystem1/2(Done) -> Sum/2
  Subsystem2/2(Done) -> Sum/3
  Switch11/1 -> Current Coord./1
  Fire/1 -> Switch11/1, Demux1/1
  Logical Operator/1 -> Memory/1, Flag1/1, Switch11/2
  Memory/1 -> Logical Operator/1

== system firefighting_drone_2/Take-off/CoordX ==
  Angular Accel : Inport
  Starting Angle : Inport  Port=2
  Desired Angle : Inport  Port=3
  If : If
  If Action Subsystem : Subsystem  TreatAsAtomicUnit=on
  If Action Subsystem1 : Subsystem  TreatAsAtomicUnit=on
  Integrator1 : Integrator
  Scope : Scope
  Scope1 : Scope
  Subsystem : Subsystem
  Sum1 : Sum  Inputs=|++
  Sum2 : Sum  Inputs=|+-
  Sum3 : Sum  Inputs=|-+
  Switch : Switch  Criteria=u2 ~= 0  SaturateOnIntegerOverflow=off  InputSameDT=off
  Out1 : Outport  VectorParamsAs1DForOutWhenUnconnected=off
  Done : Outport  Port=2  VectorParamsAs1DForOutWhenUnconnected=off
  wires:
  Angular Accel/1 -> Integrator1/1
  If Action Subsystem/1(Out1) -> Switch/3
  Sum2/1 -> If/1
  If/2 -> If Action Subsystem1/Action
  Starting Angle/1 -> Sum2/2, Sum3/2, Sum1/2
  Desired Angle/1 -> Scope1/1, Subsystem/1(Desired Angle), Sum2/1
  If Action Subsystem1/1(Out1) -> Switch/1, Switch/2
  If/1 -> If Action Subsystem/Action
  Integrator1/1 -> Sum1/1, Sum3/1
  Sum3/1 -> If Action Subsystem1/1(In1)
  Sum1/1 -> If Action Subsystem/1(In1)
  Switch/1 -> Subsystem/2(Current Angle)
  Subsystem/1(Out1) -> Scope/1, Out1/1
  Subsystem/2(Done) -> Done/1

== system firefighting_drone_2/Take-off/CoordY ==
  Angular Accel : Inport
  Starting Angle : Inport  Port=2
  Desired Angle : Inport  Port=3
  If : If
  If Action Subsystem : Subsystem  TreatAsAtomicUnit=on
  If Action Subsystem1 : Subsystem  TreatAsAtomicUnit=on
  Integrator1 : Integrator
  Scope : Scope
  Subsystem : Subsystem
  Sum1 : Sum  Inputs=|++
  Sum2 : Sum  Inputs=|+-
  Sum3 : Sum  Inputs=|-+
  Switch : Switch  Criteria=u2 ~= 0  SaturateOnIntegerOverflow=off  InputSameDT=off
  Out1 : Outport  VectorParamsAs1DForOutWhenUnconnected=off
  Done : Outport  Port=2  VectorParamsAs1DForOutWhenUnconnected=off
  wires:
  Angular Accel/1 -> Integrator1/1
  If Action Subsystem/1(Out1) -> Switch/3
  Sum2/1 -> If/1
  If/2 -> If Action Subsystem1/Action
  Starting Angle/1 -> Sum2/2, Sum3/2, Sum1/2
  Desired Angle/1 -> Subsystem/1(Desired Angle), Sum2/1
  If Action Subsystem1/1(Out1) -> Switch/1, Switch/2
  If/1 -> If Action Subsystem/Action
  Integrator1/1 -> Sum1/1, Sum3/1
  Sum3/1 -> If Action Subsystem1/1(In1)
  Sum1/1 -> If Action Subsystem/1(In1)
  Switch/1 -> Subsystem/2(Current Angle)
  Subsystem/1(Out1) -> Scope/1, Out1/1
  Subsystem/2(Done) -> Done/1

== system firefighting_drone_2/Take-off/CoordZ ==
  Angular Accel : Inport
  Starting Angle : Inport  Port=2
  Desired Angle : Inport  Port=3
  If : If
  If Action Subsystem : Subsystem  TreatAsAtomicUnit=on
  If Action Subsystem1 : Subsystem  TreatAsAtomicUnit=on
  Integrator1 : Integrator
  Scope : Scope
  Subsystem : Subsystem
  Sum1 : Sum  Inputs=|++
  Sum2 : Sum  Inputs=|+-
  Sum3 : Sum  Inputs=|-+
  Switch : Switch  Criteria=u2 ~= 0  SaturateOnIntegerOverflow=off  InputSameDT=off
  Out1 : Outport  VectorParamsAs1DForOutWhenUnconnected=off
  Done : Outport  Port=2  VectorParamsAs1DForOutWhenUnconnected=off
  wires:
  Angular Accel/1 -> Integrator1/1
  If Action Subsystem/1(Out1) -> Switch/3
  Sum2/1 -> If/1
  If/2 -> If Action Subsystem1/Action
  Starting Angle/1 -> Sum2/2, Sum3/2, Sum1/2
  Desired Angle/1 -> Subsystem/1(Desired Angle), Sum2/1
  If Action Subsystem1/1(Out1) -> Switch/1, Switch/2
  If/1 -> If Action Subsystem/Action
  Integrator1/1 -> Sum1/1, Sum3/1
  Sum3/1 -> If Action Subsystem1/1(In1)
  Sum1/1 -> If Action Subsystem/1(In1)
  Switch/1 -> Subsystem/2(Current Angle)
  Subsystem/1(Out1) -> Scope/1, Out1/1
  Subsystem/2(Done) -> Done/1

== system firefighting_drone_2/Take-off/Take-off Height ==
  Building.x : Constant  Value=0
  Building.y : Constant  Value=0
  Building.z : Constant  Value=2
  Mux : Mux  Inputs=3
  Coord : Outport  VectorParamsAs1DForOutWhenUnconnected=off
  wires:
  Building.y/1 -> Mux/2
  Building.z/1 -> Mux/3
  Building.x/1 -> Mux/1
  Mux/1 -> Coord/1

== system firefighting_drone_2/Water Tank Checks/If Action Subsystem ==
  In1 : Inport
  Action Port : ActionPort  ActionPortLabel=if(u1 > 15)
  Out1 : Outport
  wires:
  In1/1 -> Out1/1

== system firefighting_drone_2/Water Tank Checks/If Action Subsystem1 ==
  In1 : Inport
  Action Port : ActionPort  ActionPortLabel=else
  Out1 : Outport
  wires:
  In1/1 -> Out1/1

== system firefighting_drone_2/Land/Move Arm1/If Action Subsystem ==
  In1 : Inport
  Action Port : ActionPort  ActionPortLabel=if(u1 > 0)
  Out1 : Outport  VectorParamsAs1DForOutWhenUnconnected=off
  wires:
  In1/1 -> Out1/1

== system firefighting_drone_2/Land/Move Arm1/If Action Subsystem1 ==
  In1 : Inport
  Action Port : ActionPort  ActionPortLabel=else
  Out1 : Outport  VectorParamsAs1DForOutWhenUnconnected=off
  wires:
  In1/1 -> Out1/1

== system firefighting_drone_2/Land/Move Arm1/Subsystem ==
  Desired Angle : Inport
  Current Angle : Inport  Port=2
  Abs : Abs  SaturateOnIntegerOverflow=off
  Constant : Constant
  Logical Operator : Logic  Operator=OR  AllPortsSameDT=off  OutDataTypeStr=boolean
  Memory : Memory
  Relational Operator : RelationalOperator  Operator=<=  OutDataTypeStr=boolean  RndMeth=Simplest  InputSameDT=off
  Scope : Scope
  Scope1 : Scope
  Sum : Sum  Inputs=|+-
  Switch1 : Switch  Criteria=u2 > Threshold  SaturateOnIntegerOverflow=off  InputSameDT=off
  Out1 : Outport  VectorParamsAs1DForOutWhenUnconnected=off
  Done : Outport  Port=2  VectorParamsAs1DForOutWhenUnconnected=off
  wires:
  Switch1/1 -> Out1/1
  Desired Angle/1 -> Scope/1, Sum/1, Switch1/1
  Current Angle/1 -> Scope1/1, Switch1/3, Sum/2
  Sum/1 -> Abs/1
  Abs/1 -> Relational Operator/1
  Constant/1 -> Relational Operator/2
  Relational Operator/1 -> Logical Operator/2
  Logical Operator/1 -> Memory/1, Done/1, Switch1/2
  Memory/1 -> Logical Operator/1

== system firefighting_drone_2/Land/Move Arm2/If Action Subsystem ==
  In1 : Inport
  Action Port : ActionPort  ActionPortLabel=if(u1 > 0)
  Out1 : Outport  VectorParamsAs1DForOutWhenUnconnected=off
  wires:
  In1/1 -> Out1/1

== system firefighting_drone_2/Land/Move Arm2/If Action Subsystem1 ==
  In1 : Inport
  Action Port : ActionPort  ActionPortLabel=else
  Out1 : Outport  VectorParamsAs1DForOutWhenUnconnected=off
  wires:
  In1/1 -> Out1/1

== system firefighting_drone_2/Land/Move Arm2/Subsystem ==
  Desired Angle : Inport
  Current Angle : Inport  Port=2
  Abs : Abs  SaturateOnIntegerOverflow=off
  Constant : Constant
  Logical Operator : Logic  Operator=OR  AllPortsSameDT=off  OutDataTypeStr=boolean
  Memory : Memory
  Relational Operator : RelationalOperator  Operator=<=  OutDataTypeStr=boolean  RndMeth=Simplest  InputSameDT=off
  Sum : Sum  Inputs=|+-
  Switch1 : Switch  Criteria=u2 > Threshold  SaturateOnIntegerOverflow=off  InputSameDT=off
  Out1 : Outport  VectorParamsAs1DForOutWhenUnconnected=off
  Done : Outport  Port=2  VectorParamsAs1DForOutWhenUnconnected=off
  wires:
  Switch1/1 -> Out1/1
  Desired Angle/1 -> Sum/1, Switch1/1
  Current Angle/1 -> Switch1/3, Sum/2
  Sum/1 -> Abs/1
  Abs/1 -> Relational Operator/1
  Constant/1 -> Relational Operator/2
  Relational Operator/1 -> Logical Operator/2
  Logical Operator/1 -> Memory/1, Done/1, Switch1/2
  Memory/1 -> Logical Operator/1

== system firefighting_drone_2/Land/Move Arm3/If Action Subsystem ==
  In1 : Inport
  Action Port : ActionPort  ActionPortLabel=if(u1 > 0)
  Out1 : Outport  VectorParamsAs1DForOutWhenUnconnected=off
  wires:
  In1/1 -> Out1/1

== system firefighting_drone_2/Land/Move Arm3/If Action Subsystem1 ==
  In1 : Inport
  Action Port : ActionPort  ActionPortLabel=else
  Out1 : Outport  VectorParamsAs1DForOutWhenUnconnected=off
  wires:
  In1/1 -> Out1/1

== system firefighting_drone_2/Land/Move Arm3/Subsystem ==
  Desired Angle : Inport
  Current Angle : Inport  Port=2
  Abs : Abs  SaturateOnIntegerOverflow=off
  Constant : Constant
  Logical Operator : Logic  Operator=OR  AllPortsSameDT=off  OutDataTypeStr=boolean
  Memory : Memory
  Relational Operator : RelationalOperator  Operator=<=  OutDataTypeStr=boolean  RndMeth=Simplest  InputSameDT=off
  Sum : Sum  Inputs=|+-
  Switch1 : Switch  Criteria=u2 > Threshold  SaturateOnIntegerOverflow=off  InputSameDT=off
  Out1 : Outport  VectorParamsAs1DForOutWhenUnconnected=off
  Done : Outport  Port=2  VectorParamsAs1DForOutWhenUnconnected=off
  wires:
  Switch1/1 -> Out1/1
  Desired Angle/1 -> Sum/1, Switch1/1
  Current Angle/1 -> Switch1/3, Sum/2
  Sum/1 -> Abs/1
  Abs/1 -> Relational Operator/1
  Constant/1 -> Relational Operator/2
  Relational Operator/1 -> Logical Operator/2
  Logical Operator/1 -> Memory/1, Done/1, Switch1/2
  Memory/1 -> Logical Operator/1

== system firefighting_drone_2/Move To Home/Move Arm1/If Action Subsystem ==
  In1 : Inport
  Action Port : ActionPort  ActionPortLabel=if(u1 > 0)
  Out1 : Outport  VectorParamsAs1DForOutWhenUnconnected=off
  wires:
  In1/1 -> Out1/1

== system firefighting_drone_2/Move To Home/Move Arm1/If Action Subsystem1 ==
  In1 : Inport
  Action Port : ActionPort  ActionPortLabel=else
  Out1 : Outport  VectorParamsAs1DForOutWhenUnconnected=off
  wires:
  In1/1 -> Out1/1

== system firefighting_drone_2/Move To Home/Move Arm1/Subsystem ==
  Desired Angle : Inport
  Current Angle : Inport  Port=2
  Abs : Abs  SaturateOnIntegerOverflow=off
  Constant : Constant
  Logical Operator : Logic  Operator=OR  AllPortsSameDT=off  OutDataTypeStr=boolean
  Memory : Memory
  Relational Operator : RelationalOperator  Operator=<=  OutDataTypeStr=boolean  RndMeth=Simplest  InputSameDT=off
  Scope : Scope
  Scope1 : Scope
  Sum : Sum  Inputs=|+-
  Switch1 : Switch  Criteria=u2 > Threshold  SaturateOnIntegerOverflow=off  InputSameDT=off
  Out1 : Outport  VectorParamsAs1DForOutWhenUnconnected=off
  Done : Outport  Port=2  VectorParamsAs1DForOutWhenUnconnected=off
  wires:
  Switch1/1 -> Out1/1
  Desired Angle/1 -> Scope/1, Sum/1, Switch1/1
  Current Angle/1 -> Scope1/1, Switch1/3, Sum/2
  Sum/1 -> Abs/1
  Abs/1 -> Relational Operator/1
  Constant/1 -> Relational Operator/2
  Relational Operator/1 -> Logical Operator/2
  Logical Operator/1 -> Memory/1, Done/1, Switch1/2
  Memory/1 -> Logical Operator/1

== system firefighting_drone_2/Move To Home/Move Arm2/If Action Subsystem ==
  In1 : Inport
  Action Port : ActionPort  ActionPortLabel=if(u1 > 0)
  Out1 : Outport  VectorParamsAs1DForOutWhenUnconnected=off
  wires:
  In1/1 -> Out1/1

== system firefighting_drone_2/Move To Home/Move Arm2/If Action Subsystem1 ==
  In1 : Inport
  Action Port : ActionPort  ActionPortLabel=else
  Out1 : Outport  VectorParamsAs1DForOutWhenUnconnected=off
  wires:
  In1/1 -> Out1/1

== system firefighting_drone_2/Move To Home/Move Arm2/Subsystem ==
  Desired Angle : Inport
  Current Angle : Inport  Port=2
  Abs : Abs  SaturateOnIntegerOverflow=off
  Constant : Constant
  Logical Operator : Logic  Operator=OR  AllPortsSameDT=off  OutDataTypeStr=boolean
  Memory : Memory
  Relational Operator : RelationalOperator  Operator=<=  OutDataTypeStr=boolean  RndMeth=Simplest  InputSameDT=off
  Sum : Sum  Inputs=|+-
  Switch1 : Switch  Criteria=u2 > Threshold  SaturateOnIntegerOverflow=off  InputSameDT=off
  Out1 : Outport  VectorParamsAs1DForOutWhenUnconnected=off
  Done : Outport  Port=2  VectorParamsAs1DForOutWhenUnconnected=off
  wires:
  Switch1/1 -> Out1/1
  Desired Angle/1 -> Sum/1, Switch1/1
  Current Angle/1 -> Switch1/3, Sum/2
  Sum/1 -> Abs/1
  Abs/1 -> Relational Operator/1
  Constant/1 -> Relational Operator/2
  Relational Operator/1 -> Logical Operator/2
  Logical Operator/1 -> Memory/1, Done/1, Switch1/2
  Memory/1 -> Logical Operator/1

== system firefighting_drone_2/Move To Home/Move Arm3/If Action Subsystem ==
  In1 : Inport
  Action Port : ActionPort  ActionPortLabel=if(u1 > 0)
  Out1 : Outport  VectorParamsAs1DForOutWhenUnconnected=off
  wires:
  In1/1 -> Out1/1

== system firefighting_drone_2/Move To Home/Move Arm3/If Action Subsystem1 ==
  In1 : Inport
  Action Port : ActionPort  ActionPortLabel=else
  Out1 : Outport  VectorParamsAs1DForOutWhenUnconnected=off
  wires:
  In1/1 -> Out1/1

== system firefighting_drone_2/Move To Home/Move Arm3/Subsystem ==
  Desired Angle : Inport
  Current Angle : Inport  Port=2
  Abs : Abs  SaturateOnIntegerOverflow=off
  Constant : Constant
  Logical Operator : Logic  Operator=OR  AllPortsSameDT=off  OutDataTypeStr=boolean
  Memory : Memory
  Relational Operator : RelationalOperator  Operator=<=  OutDataTypeStr=boolean  RndMeth=Simplest  InputSameDT=off
  Sum : Sum  Inputs=|+-
  Switch1 : Switch  Criteria=u2 > Threshold  SaturateOnIntegerOverflow=off  InputSameDT=off
  Out1 : Outport  VectorParamsAs1DForOutWhenUnconnected=off
  Done : Outport  Port=2  VectorParamsAs1DForOutWhenUnconnected=off
  wires:
  Switch1/1 -> Out1/1
  Desired Angle/1 -> Sum/1, Switch1/1
  Current Angle/1 -> Switch1/3, Sum/2
  Sum/1 -> Abs/1
  Abs/1 -> Relational Operator/1
  Constant/1 -> Relational Operator/2
  Relational Operator/1 -> Logical Operator/2
  Logical Operator/1 -> Memory/1, Done/1, Switch1/2
  Memory/1 -> Logical Operator/1

== system firefighting_drone_2/Move To Waypoint/Move X/If Action Subsystem ==
  In1 : Inport
  Action Port : ActionPort  ActionPortLabel=if(u1 > 0)
  Out1 : Outport  VectorParamsAs1DForOutWhenUnconnected=off
  wires:
  In1/1 -> Out1/1

== system firefighting_drone_2/Move To Waypoint/Move X/If Action Subsystem1 ==
  In1 : Inport
  Action Port : ActionPort  ActionPortLabel=else
  Out1 : Outport  VectorParamsAs1DForOutWhenUnconnected=off
  wires:
  In1/1 -> Out1/1

== system firefighting_drone_2/Move To Waypoint/Move X/Subsystem ==
  Desired Angle : Inport
  Current Angle : Inport  Port=2
  Abs : Abs  SaturateOnIntegerOverflow=off
  Constant : Constant
  Logical Operator : Logic  Operator=OR  AllPortsSameDT=off  OutDataTypeStr=boolean
  Memory : Memory
  Relational Operator : RelationalOperator  Operator=<=  OutDataTypeStr=boolean  RndMeth=Simplest  InputSameDT=off
  Scope : Scope
  Scope1 : Scope
  Sum : Sum  Inputs=|+-
  Switch1 : Switch  Criteria=u2 > Threshold  SaturateOnIntegerOverflow=off  InputSameDT=off
  Out1 : Outport  VectorParamsAs1DForOutWhenUnconnected=off
  Done : Outport  Port=2  VectorParamsAs1DForOutWhenUnconnected=off
  wires:
  Switch1/1 -> Out1/1
  Desired Angle/1 -> Scope/1, Sum/1, Switch1/1
  Current Angle/1 -> Scope1/1, Switch1/3, Sum/2
  Sum/1 -> Abs/1
  Abs/1 -> Relational Operator/1
  Constant/1 -> Relational Operator/2
  Relational Operator/1 -> Logical Operator/2
  Logical Operator/1 -> Memory/1, Done/1, Switch1/2
  Memory/1 -> Logical Operator/1

== system firefighting_drone_2/Move To Waypoint/Move Y/If Action Subsystem ==
  In1 : Inport
  Action Port : ActionPort  ActionPortLabel=if(u1 > 0)
  Out1 : Outport  VectorParamsAs1DForOutWhenUnconnected=off
  wires:
  In1/1 -> Out1/1

== system firefighting_drone_2/Move To Waypoint/Move Y/If Action Subsystem1 ==
  In1 : Inport
  Action Port : ActionPort  ActionPortLabel=else
  Out1 : Outport  VectorParamsAs1DForOutWhenUnconnected=off
  wires:
  In1/1 -> Out1/1

== system firefighting_drone_2/Move To Waypoint/Move Y/Subsystem ==
  Desired Angle : Inport
  Current Angle : Inport  Port=2
  Abs : Abs  SaturateOnIntegerOverflow=off
  Constant : Constant
  Logical Operator : Logic  Operator=OR  AllPortsSameDT=off  OutDataTypeStr=boolean
  Memory : Memory
  Relational Operator : RelationalOperator  Operator=<=  OutDataTypeStr=boolean  RndMeth=Simplest  InputSameDT=off
  Sum : Sum  Inputs=|+-
  Switch1 : Switch  Criteria=u2 > Threshold  SaturateOnIntegerOverflow=off  InputSameDT=off
  Out1 : Outport  VectorParamsAs1DForOutWhenUnconnected=off
  Done : Outport  Port=2  VectorParamsAs1DForOutWhenUnconnected=off
  wires:
  Switch1/1 -> Out1/1
  Desired Angle/1 -> Sum/1, Switch1/1
  Current Angle/1 -> Switch1/3, Sum/2
  Sum/1 -> Abs/1
  Abs/1 -> Relational Operator/1
  Constant/1 -> Relational Operator/2
  Relational Operator/1 -> Logical Operator/2
  Logical Operator/1 -> Memory/1, Done/1, Switch1/2
  Memory/1 -> Logical Operator/1

== system firefighting_drone_2/Move To Waypoint/Move Z/If Action Subsystem ==
  In1 : Inport
  Action Port : ActionPort  ActionPortLabel=if(u1 > 0)
  Out1 : Outport  VectorParamsAs1DForOutWhenUnconnected=off
  wires:
  In1/1 -> Out1/1

== system firefighting_drone_2/Move To Waypoint/Move Z/If Action Subsystem1 ==
  In1 : Inport
  Action Port : ActionPort  ActionPortLabel=else
  Out1 : Outport  VectorParamsAs1DForOutWhenUnconnected=off
  wires:
  In1/1 -> Out1/1

== system firefighting_drone_2/Move To Waypoint/Move Z/Subsystem ==
  Desired Angle : Inport
  Current Angle : Inport  Port=2
  Abs : Abs  SaturateOnIntegerOverflow=off
  Constant : Constant
  Logical Operator : Logic  Operator=OR  AllPortsSameDT=off  OutDataTypeStr=boolean
  Memory : Memory
  Relational Operator : RelationalOperator  Operator=<=  OutDataTypeStr=boolean  RndMeth=Simplest  InputSameDT=off
  Sum : Sum  Inputs=|+-
  Switch1 : Switch  Criteria=u2 > Threshold  SaturateOnIntegerOverflow=off  InputSameDT=off
  Out1 : Outport  VectorParamsAs1DForOutWhenUnconnected=off
  Done : Outport  Port=2  VectorParamsAs1DForOutWhenUnconnected=off
  wires:
  Switch1/1 -> Out1/1
  Desired Angle/1 -> Sum/1, Switch1/1
  Current Angle/1 -> Switch1/3, Sum/2
  Sum/1 -> Abs/1
  Abs/1 -> Relational Operator/1
  Constant/1 -> Relational Operator/2
  Relational Operator/1 -> Logical Operator/2
  Logical Operator/1 -> Memory/1, Done/1, Switch1/2
  Memory/1 -> Logical Operator/1

== system firefighting_drone_2/Search for Fire/Seaerch-fire/B1 ==
  Building : Inport
  Constant : Constant  Value=18
  Demux : Demux  Outputs=3
  Mux : Mux  Inputs=3
  Sum : Sum  Inputs=|++
  O : Outport  VectorParamsAs1DForOutWhenUnconnected=off
  wires:
  Mux/1 -> O/1
  Demux/3 -> Sum/1
  Constant/1 -> Sum/2
  Sum/1 -> Mux/3
  Building/1 -> Demux/1
  Demux/1 -> Mux/1
  Demux/2 -> Mux/2

== system firefighting_drone_2/Search for Fire/Seaerch-fire/B10 ==
  In1 : Inport
  Constant : Constant  Value=2
  Demux : Demux  Outputs=3
  Mux : Mux  Inputs=3
  Sum : Sum  Inputs=|++
  O : Outport  VectorParamsAs1DForOutWhenUnconnected=off
  wires:
  Mux/1 -> O/1
  Constant/1 -> Sum/2
  In1/1 -> Demux/1
  Demux/1 -> Mux/1
  Demux/2 -> Sum/1
  Sum/1 -> Mux/2
  Demux/3 -> Mux/3

== system firefighting_drone_2/Search for Fire/Seaerch-fire/B11 ==
  In1 : Inport
  In2 : Inport  Port=2
  Constant : Constant  Value=18
  Demux : Demux  Outputs=3
  Mux : Mux  Inputs=3
  Sum : Sum  Inputs=|+-
  O : Outport  VectorParamsAs1DForOutWhenUnconnected=off
  wires:
  Mux/1 -> O/1
  Demux/3 -> Sum/1
  Constant/1 -> Sum/2
  Sum/1 -> Mux/3
  In1/1 -> Demux/1
  Demux/1 -> Mux/1
  Demux/2 -> Mux/2

== system firefighting_drone_2/Search for Fire/Seaerch-fire/B2 ==
  In1 : Inport
  Constant : Constant  Value=2
  Demux : Demux  Outputs=3
  Mux : Mux  Inputs=3
  Sum : Sum  Inputs=|++
  O : Outport  VectorParamsAs1DForOutWhenUnconnected=off
  wires:
  Mux/1 -> O/1
  Constant/1 -> Sum/2
  In1/1 -> Demux/1
  Demux/1 -> Mux/1
  Demux/2 -> Sum/1
  Sum/1 -> Mux/2
  Demux/3 -> Mux/3

== system firefighting_drone_2/Search for Fire/Seaerch-fire/B3 ==
  In1 : Inport
  Constant : Constant  Value=18
  Demux : Demux  Outputs=3
  Mux : Mux  Inputs=3
  Sum : Sum  Inputs=|+-
  O : Outport  VectorParamsAs1DForOutWhenUnconnected=off
  wires:
  Mux/1 -> O/1
  Demux/3 -> Sum/1
  Constant/1 -> Sum/2
  Sum/1 -> Mux/3
  In1/1 -> Demux/1
  Demux/1 -> Mux/1
  Demux/2 -> Mux/2
